simulink model "CONTROL_STARTER_2018b"  (R2018b)
settings: Solver=VariableStepAuto  StartTime=0.0  StopTime=10.0  RelTol=1e-3
settings Model: Creator=EGI-Z400  LastModifiedBy=HWRL user
settings DataIOCC: ReturnWorkspaceOutputs=on
settings DebuggingCC: SFMachineParentedDataDiag=error

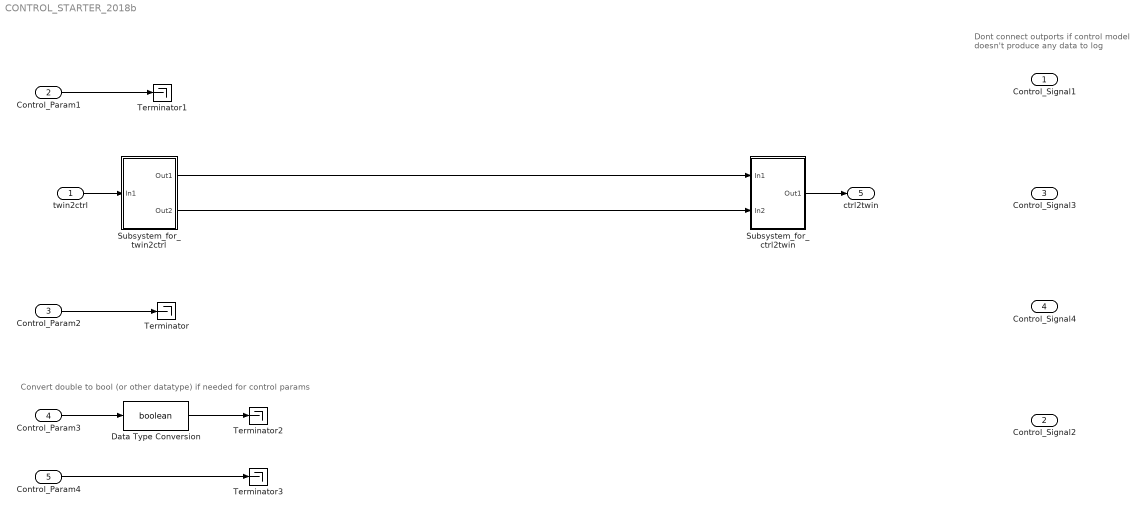
== system CONTROL_STARTER_2018b ==
  note: Convert double to bool (or other datatype) if needed for control params
  note: Dont connect outports if control
      | model doesn't produce any data
      | to log
  twin2ctrl : Inport
  Control_Param1 : Inport  Port=2
  Control_Param2 : Inport  Port=3
  Control_Param3 : Inport  Port=4  OutDataTypeStr=double
  Control_Param4 : Inport  Port=5  OutDataTypeStr=double
  Data Type Conversion : DataTypeConversion  OutDataTypeStr=boolean
  Subsystem_for_ctrl2twin : Subsystem
  Subsystem_for_twin2ctrl : Subsystem
  Terminator{,1..3} (4 alike) : Terminator
  Control_Signal1 : Outport
  Control_Signal2 : Outport  Port=2
  Control_Signal3 : Outport  Port=3
  Control_Signal4 : Outport  Port=4
  ctrl2twin : Outport  Port=5
  wires:
  Control_Param3/1 -> Data Type Conversion/1
  Control_Param4/1 -> Terminator3/1
  Control_Param2/1 -> Terminator/1
  Control_Param1/1 -> Terminator1/1
  Data Type Conversion/1 -> Terminator2/1
  twin2ctrl/1 -> Subsystem_for_twin2ctrl/1(In1)
  Subsystem_for_ctrl2twin/1(Out1) -> ctrl2twin/1
  Subsystem_for_twin2ctrl/1(Out1) -> Subsystem_for_ctrl2twin/1(In1)
  Subsystem_for_twin2ctrl/2(Out2) -> Subsystem_for_ctrl2twin/2(In2)

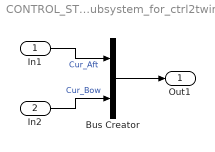
== system CONTROL_STARTER_2018b/Subsystem_for_ctrl2twin ==
  In1 : Inport
  In2 : Inport  Port=2
  Bus Creator : BusCreator  Inputs=2
  Out1 : Outport
  wires:
  In1/1 -> Bus Creator/1  "Cur_Aft"
  In2/1 -> Bus Creator/2  "Cur_Bow"
  Bus Creator/1 -> Out1/1

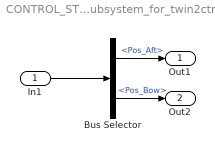
== system CONTROL_STARTER_2018b/Subsystem_for_twin2ctrl ==
  In1 : Inport
  Bus Selector : BusSelector  OutputSignals=Pos_Aft,Pos_Bow
  Out1 : Outport
  Out2 : Outport  Port=2
  wires:
  In1/1 -> Bus Selector/1
  Bus Selector/1 -> Out1/1  "<Pos_Aft>"
  Bus Selector/2 -> Out2/1  "<Pos_Bow>"
